simulink model "Logical"  (R2017b)
settings: Solver=FixedStepDiscrete  StartTime=0.0  StopTime=10.0  FixedStep=0.200000  RelTol=1e-3  EnableMultiTasking=on
model workspace (MAT data in the model file):
  already_pp = 0
  input_struct.time = [0; 0.2; 0.4; 0.6; 0.8; 1; 1.2; 1.4; 1.6; 1.8; 2; 2.2; 2.4; 2.6; 2.8; 3; 3.2; 3.4; 3.6; 3.8; 4; 4.2; 4.4; 4.6; 4.8; 5; 5.2; 5.4; 5.6; 5.8; 6; 6.2; 6.4; 6.6; 6.8; 7; 7.2; 7.4; 7.6; 7.8; 8; 8.2; 8.4; 8.6; 8.8; 9; 9.2; 9.4; 9.6; 9.8; 10; 10.2; 10.4; 10.6; 10.8; 11; 11.2; 11.4; 11.6; 11.8; 12; 12.2; 12.4; 12.6; 12.8; 13; 13.2; 13.4; 13.6; 13.8; 14; 14.2; 14.4; 14.6; 14.8; 15; 15.2; 15.4; 15.6; 15.8; 16; 16.2; 16.4; 16.6; 16.8; 17; 17.2; 17.4; 17.6; 17.8; 18; 18.2; 18.4; 18.6; 18.8; 19; 19.2; 19.4; 19.6; 19.8]
  input_struct.signals(1).name = 'In4'
  input_struct.signals(1).values = [23.1846467113 23.6830652766 78.8570257461 55.4734347792 85.9555655331 36.0820456969 45.4949694914 74.5835903343 46.1757001113 46.6711602877 9.78869943206 1.67411285472 ... (300 elements, 100x3)]
  input_struct.signals(1).dimensions = 3
  input_struct.signals(2).name = 'In1'
  input_struct.signals(2).values = [46  20  25; 78  90  71; 24  59  24; 31  88  61; 94  45  10; 47  80  91; 24  32  51; 9  3  63; 45  11  68; 46  32  29; 89  16  36; 97  41  14; 37  81  55; 99  42  24; 9  56  53; 9  69  97; 95  86  1; 71  85  46; 68  40  74; 48  5  89; 15  22  90; 73  53  63; 2  82  67; 84  75  76; 90  23  65; 15  61  49; 11  82  17; 3  9  56; 24  77  66; 87  24  16; 30  7  83; 88  9  48; 66  29  6; 56  22  10; 91  15  26; 51  58  17; 97  18  44; 44  1  1; 32  1  11; 10  50  82; 80  29  40; 85  53  11; 62  94  96; 9  30  2; 27  12  49; 22  77  18; 32  60  93; 29  50  5; 45  39  83; 96  28  77; 39  27  28; 7  75  85; 92  90  65; 55  92  73; 29  47  40; 53  76  24; 97  62  92; 71  62  44; 95  61  70; 25  35  7; 57  55  87; 53  14  90; 86  77  97; 38  66  79; 94  55  19; 2  81  18; 59  12  30; 54  14  31; 20  79  2; 6  86  89; 15  15  79; 2  66  38; 61  52  64; 56  1  81; 60  70  7; 23  77  88; 83  51  95; 30  92  14; 7  16  62; 27  23  15; 90  1  91; 35  82  67; 15  94  9; 64  9  8; 65  65  91; 91  11  20; 38  64  22; 74  30  68; 49  89  54; 95  35  42; 90  74  9; 17  100  49; 85  10  38; 84  45  26; 48  28  69; 88  72  16; 84  10  93; 30  6  63; 6  74  80; 7  24  7]
  input_struct.signals(2).dimensions = 3
  input_struct.signals(3).name = 'In2'
  input_struct.signals(3).values = [16.8206021447 92.2505104099 75.9487435631 28.5920916432 91.7213188604 4.1027655719 54.8577754154 75.2552668021 49.3286034243 40.3682180693 6.32908979548 32.6320786865 ... (300 elements, 100x3)]
  input_struct.signals(3).dimensions = 3
  input_struct.signals(4).name = 'In3'
  input_struct.signals(4).values = [47.0994932453 59.2500151649 42.6508590108 15.3168974514 24.4819400571 49.604814842 95.5594586597 11.9394050937 52.2687214044 23.2806260184 95.1363309642 19.1147017959 ... (300 elements, 100x3)]
  input_struct.signals(4).dimensions = 3
  input_struct.signals(5).name = 'In5'
  input_struct.signals(5).values = [7.77472195615 2.6099025129 77.3013609893 67.6912852716 13.1921651761 77.3024970161 10.8010416764 45.3606052435 68.8337979254 79.3347560771 27.3731954601 6.33665699807 ... (300 elements, 100x3)]
  input_struct.signals(5).dimensions = 3
  input_struct.signals(6).name = 'In6'
  input_struct.signals(6).values = [61.3266670144 95.3120716737 65.1433922039 11.7649230247 63.1742640243 58.5341434164 14.0663615941 72.594145636 48.5340563371 45.986640117 44.1010757039 6.9633923325 ... (300 elements, 100x3)]
  input_struct.signals(6).dimensions = 3
  input_struct.signals(7).name = 'In7'
  input_struct.signals(7).values = [89.296138317 82.1812861024 73.4736298852 21.023117929 56.4222425656 21.6710720562 6.17746193697 31.3839408492 42.3774899071 38.9730917055 87.9331018203 94.985766289 ... (300 elements, 100x3)]
  input_struct.signals(7).dimensions = 3
  input_struct.signals(8).name = 'In8'
  input_struct.signals(8).values = [91.8179154692 98.4564241742 30.4628234912 7.91615270124 73.5384998477 94.0767889781 52.3171176275 2.00649791533 71.4840235656 32.2462332058 33.3701856797 46.1196402977 ... (300 elements, 100x3)]
  input_struct.signals(8).dimensions = 3
  input_struct.signals(9).name = 'In9'
  input_struct.signals(9).values = [83.2190970376 17.0291191428 80.7475685434 17.920947355 22.407306588 22.7777222047 69.9266515504 49.7181601153 12.4723924658 73.5039216726 15.5630235753 91.8272170909 ... (300 elements, 100x3)]
  input_struct.signals(9).dimensions = 3
  input_struct.signals(10).name = 'In10'
  input_struct.signals(10).values = [82.6185642866 85.9301842883 28.9945949326 44.9799680665 43.8882782538 21.6602935353 92.1964984046 13.8433388719 53.8732988886 60.4721828245 33.3207482286 76.2585053899 ... (300 elements, 100x3)]
  input_struct.signals(10).dimensions = 3
  input_struct.signals(11).name = 'In11'
  input_struct.signals(11).values = [56.675547985 68.8382307995 42.7649852455 20.5599727444 78.2694602826 62.9349201486 79.7933351569 28.0636373415 45.1817772404 4.89202060838 81.8214023639 3.64728824123 ... (300 elements, 100x3)]
  input_struct.signals(11).dimensions = 3
  input_struct.signals(12).name = 'In12'
  input_struct.signals(12).values = [32.1614942647 59.2038921272 18.4123246891 51.1288201396 18.6694083543 40.7794676999 42.4090759235 94.3180045524 94.1127238142 77.4992178862 21.301771478 76.4546178791 ... (300 elements, 100x3)]
  input_struct.signals(12).dimensions = 3
  input_struct.signals(13).name = 'In13'
  input_struct.signals(13).values = [99.548945832 17.0592034793 30.1997290946 16.8681980745 7.7059358178 38.6308311921 25.8724696207 41.397959929 86.2214480483 55.6984646072 81.1671116065 19.1365102819 ... (300 elements, 100x3)]
  input_struct.signals(13).dimensions = 3
settings Model: Creator=hbourbou  LastModifiedBy=hbourbou
settings DataIOCC: SaveFormat=StructureWithTime
settings OptimizationCC: LifeSpan=inf
settings DebuggingCC: AlgebraicLoopMsg=error  ArtificialAlgebraicLoopMsg=error  SFExecutionAtInitializationDiag=none
settings HardwareCC: ProdBitPerSizeT=32  ProdBitPerPtrDiffT=32  ProdWordSize=32  ProdHWDeviceType=Specified
settings CodeAppCC: StateflowObjectComments=on

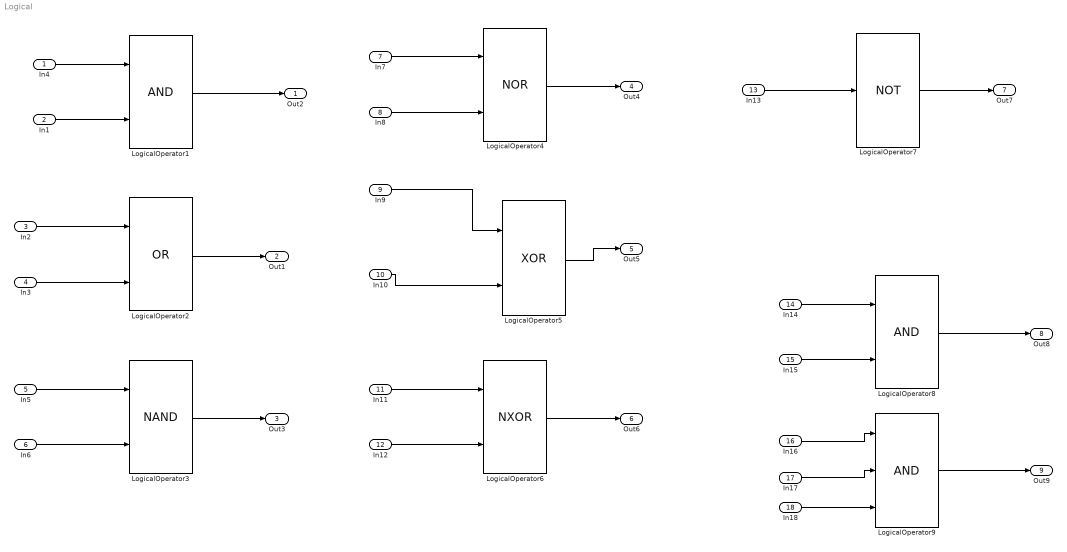
== system Logical ==
  In4 : Inport  OutDataTypeStr=double  PortDimensions=3
  In1 : Inport  Port=2  OutDataTypeStr=int8  PortDimensions=3
  In2 : Inport  Port=3  OutDataTypeStr=double  PortDimensions=3
  In3 : Inport  Port=4  OutDataTypeStr=double  PortDimensions=3
  In5 : Inport  Port=5  OutDataTypeStr=double  PortDimensions=3
  In6 : Inport  Port=6  OutDataTypeStr=double  PortDimensions=3
  In7 : Inport  Port=7  OutDataTypeStr=double  PortDimensions=3
  In8 : Inport  Port=8  OutDataTypeStr=double  PortDimensions=3
  In9 : Inport  Port=9  OutDataTypeStr=double  PortDimensions=3
  In10 : Inport  Port=10  OutDataTypeStr=double  PortDimensions=3
  In11 : Inport  Port=11  OutDataTypeStr=double  PortDimensions=3
  In12 : Inport  Port=12  OutDataTypeStr=double  PortDimensions=3
  In13 : Inport  Port=13  OutDataTypeStr=double  PortDimensions=3
  In14 : Inport  Port=14  OutDataTypeStr=double  PortDimensions=1
  In15 : Inport  Port=15  OutDataTypeStr=int8  PortDimensions=3
  In16 : Inport  Port=16  OutDataTypeStr=double  PortDimensions=1
  In17 : Inport  Port=17  OutDataTypeStr=int8  PortDimensions=3
  In18 : Inport  Port=18  OutDataTypeStr=int8  PortDimensions=3
  LogicalOperator1 : Logic  AllPortsSameDT=off  OutDataTypeStr=boolean
  LogicalOperator2 : Logic  Operator=OR  AllPortsSameDT=off  OutDataTypeStr=boolean
  LogicalOperator3 : Logic  Operator=NAND  AllPortsSameDT=off  OutDataTypeStr=boolean
  LogicalOperator4 : Logic  Operator=NOR  AllPortsSameDT=off  OutDataTypeStr=boolean
  LogicalOperator5 : Logic  Operator=XOR  AllPortsSameDT=off  OutDataTypeStr=boolean
  LogicalOperator6 : Logic  Operator=NXOR  AllPortsSameDT=off  OutDataTypeStr=boolean
  LogicalOperator7 : Logic  Operator=NOT  AllPortsSameDT=off  OutDataTypeStr=boolean
  LogicalOperator8 : Logic  AllPortsSameDT=off  OutDataTypeStr=boolean
  LogicalOperator9 : Logic  Inputs=3  AllPortsSameDT=off  OutDataTypeStr=boolean
  Out2 : Outport
  Out1 : Outport  Port=2
  Out3 : Outport  Port=3
  Out4 : Outport  Port=4
  Out5 : Outport  Port=5
  Out6 : Outport  Port=6
  Out7 : Outport  Port=7
  Out8 : Outport  Port=8
  Out9 : Outport  Port=9
  wires:
  LogicalOperator1/1 -> Out2/1
  In4/1 -> LogicalOperator1/1
  In1/1 -> LogicalOperator1/2
  LogicalOperator2/1 -> Out1/1
  In2/1 -> LogicalOperator2/1
  In3/1 -> LogicalOperator2/2
  LogicalOperator3/1 -> Out3/1
  In5/1 -> LogicalOperator3/1
  In6/1 -> LogicalOperator3/2
  LogicalOperator4/1 -> Out4/1
  In7/1 -> LogicalOperator4/1
  In8/1 -> LogicalOperator4/2
  LogicalOperator5/1 -> Out5/1
  In9/1 -> LogicalOperator5/1
  In10/1 -> LogicalOperator5/2
  LogicalOperator6/1 -> Out6/1
  In11/1 -> LogicalOperator6/1
  In12/1 -> LogicalOperator6/2
  LogicalOperator7/1 -> Out7/1
  In13/1 -> LogicalOperator7/1
  LogicalOperator8/1 -> Out8/1
  In14/1 -> LogicalOperator8/1
  In15/1 -> LogicalOperator8/2
  LogicalOperator9/1 -> Out9/1
  In16/1 -> LogicalOperator9/1
  In17/1 -> LogicalOperator9/2
  In18/1 -> LogicalOperator9/3
